simulink model "controllo_ss_PP_Luenberger"  (R2023b)
settings: Solver=VariableStepAuto  StartTime=0.0  StopTime=5  RelTol=1e-3
values from neighbouring files (symbols this model uses):
  A_ob = A - L_kf*C    [LQ_KF.m]    (also in LQ_KF_version1.m; LQ_KF_version2.m; LQ_Luenberger.m = A - L*C; LQ_prova.m)
  B_ob = [ B - L_kf*D, L_kf]    [LQ_KF.m]    (also in LQ_KF_version1.m; LQ_KF_version2.m; LQ_Luenberger.m = [ B - L*D, L]; LQ_prova.m)
  C_ob = eye(n)    [LQ_KF.m]    (also in LQ_KF_version1.m; LQ_KF_version2.m; LQ_Luenberger.m; LQ_prova.m)
  D_ob = zeros(n, m+p)    [LQ_KF.m]    (also in LQ_KF_version1.m; LQ_KF_version2.m; LQ_Luenberger.m; LQ_prova.m)
  Ken_eta = K(:, 4)    [LQ_KF.m]    (also in LQ_KF_version1.m; LQ_KF_version2.m = Ken(:, n+1:end); LQ_Luenberger.m; LQ_prova.m = Ken(:, n+1:end))
  Ken_x = K(:, 1:3)    [LQ_KF.m]    (also in LQ_KF_version1.m; LQ_KF_version2.m = Ken(:, 1:n); LQ_Luenberger.m; LQ_prova.m = Ken(:, 1:n))
undefined symbols (not defined in the file or in its folder): A, B, C, D, x1_eq0, x2_eq0
libraries: SignalEditorBlockLib x1
settings Model: Creator=Pronto all'uso  LastModifiedBy=lollo

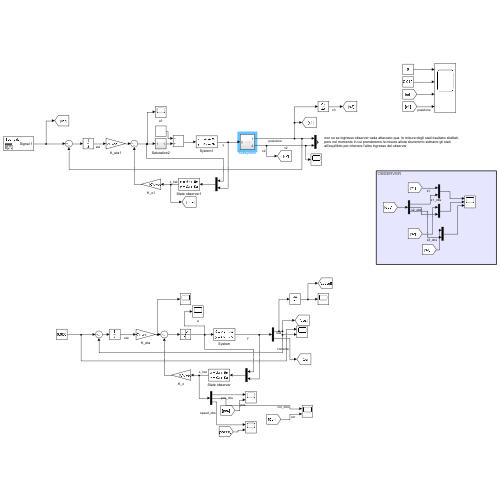
[thumbnail: Simulink's stored preview of the top-level diagram]
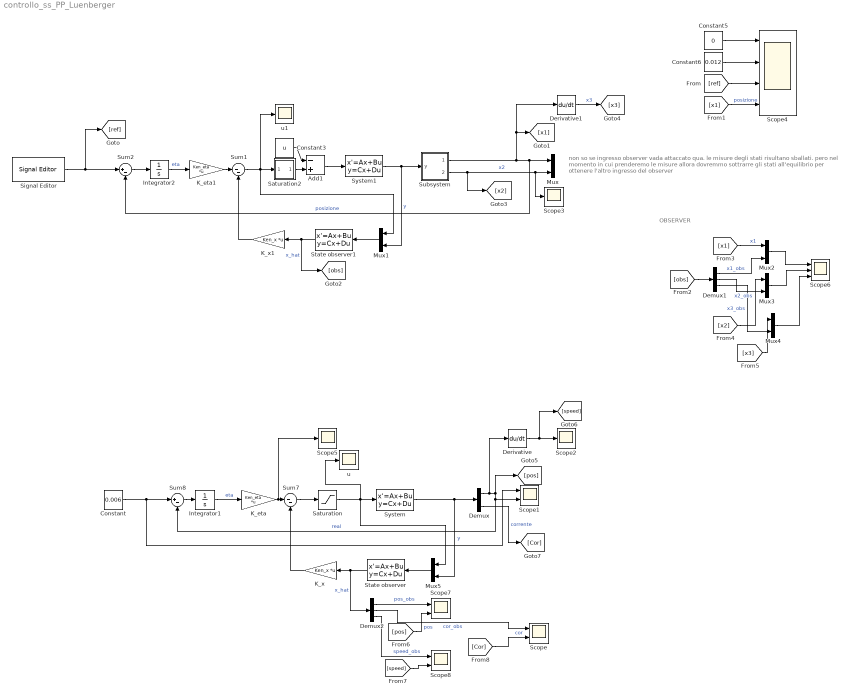
== system controllo_ss_PP_Luenberger ==
  note: OBSERVER
  note: non so se ingresso observer vada attaccato qua. le misure degli stati risultano sballati. pero nel momento in cui prenderemo le misure allora dovremmo sottrarre gli stati all'equilibrio per ottenere l'altro ingresso del observer
  Add1 : Sum  Inputs=-+
  Constant : Constant  Value=0.006
  Constant3 : Constant  Value=u
  Constant5 : Constant  Value=0
  Constant6 : Constant  Value=0.012
  Demux : Demux  Outputs=2
  Demux1 : Demux  Outputs=3
  Demux2 : Demux  Outputs=3
  Derivative : Derivative
  Derivative1 : Derivative
  Integrator1 : Integrator
  Integrator2 : Integrator
  K_eta : Gain  Gain=Ken_eta  Multiplication=Matrix(K*u) (u vector)
  K_eta1 : Gain  Gain=Ken_eta  Multiplication=Matrix(K*u) (u vector)
  K_x : Gain  Gain=Ken_x  Multiplication=Matrix(K*u) (u vector)
  K_x1 : Gain  Gain=Ken_x  Multiplication=Matrix(K*u) (u vector)
  Mux{,1..5} (6 alike) : Mux  Inputs=2
  Saturation : Saturate  UpperLimit=23  LowerLimit=-23
  Saturation2 : Subsystem
  Scope{,1,7..8} (4 alike) : Scope  NumInputPorts=2
  Scope2 : Scope
  Scope3 : Scope
  Scope4 : Scope  NumInputPorts=4
  Scope5 : Scope
  Scope6 : Scope  NumInputPorts=3
  Signal Editor : SignalEditorBlockLib/Signal Editor  FileName=input_signal.mat  ActiveScenario=Scenario  ActiveSignal=Signal 1  IsBus=off  OutputBusObjectStr=Bus: BusObject  SampleTime=0  Interpolate=off  ZeroCross=off  OutputAfterFinalValue=Setting to zero  Unit=inherit  PreserveSignalName=on  ApplySigPropsToAllScenarios=on  ApplySigPropsToAllSignals=off
  State observer : StateSpace  A=A_ob  B=B_ob  C=C_ob  D=D_ob  InitialCondition=[0.002;0;0]  ParameterTunability=Unconstrained
  State observer1 : StateSpace  A=A_ob  B=B_ob  C=C_ob  D=D_ob  InitialCondition=[0.002;0;0]  ParameterTunability=Unconstrained
  Subsystem : Subsystem
  Sum1 : Sum  Inputs=|--
  Sum2 : Sum  Inputs=|+-
  Sum7 : Sum  Inputs=|--
  Sum8 : Sum  Inputs=|+-
  System : StateSpace  A=A  B=B  C=C  D=D  InitialCondition=[0; 0;0]  ParameterTunability=Unconstrained
  System1 : StateSpace  A=A  B=B  C=C  D=D  InitialCondition=[0; 0;0]  ParameterTunability=Unconstrained
  u : Scope
  u1 : Scope
  wires:
  Integrator1/1 -> K_eta/1  "eta"
  K_x/1 -> Sum7/2
  Sum8/1 -> Integrator1/1
  K_eta/1 -> Scope5/1, Sum7/1
  System/1 -> Demux/1, Mux5/2  "y"
  State observer/1 -> Demux2/1, K_x/1  "x_hat"
  Mux5/1 -> State observer/1
  Demux/1 -> Derivative/1, [pos], Scope1/2, Sum8/2  "real"
  Demux/2 -> [Cor]  "corrente"
  Constant/1 -> Scope1/1, Sum8/1
  Sum7/1 -> Saturation/1
  Saturation/1 -> Mux5/1, u/1, System/1
  Derivative/1 -> [speed], Scope2/1
  State observer1/1 -> [obs], K_x1/1  "x_hat"
  Sum2/1 -> Integrator2/1
  Integrator2/1 -> K_eta1/1  "eta"
  Sum1/1 -> u1/1, Saturation2/1(In1), Mux1/1
  K_eta1/1 -> Sum1/1
  K_x1/1 -> Sum1/2
  Signal Editor/1 -> [ref], Sum2/1
  Mux1/1 -> State observer1/1
  [ref] -> Scope4/3
  Add1/1 -> System1/1
  Constant3/1 -> Add1/1
  Constant5/1 -> Scope4/1
  Constant6/1 -> Scope4/2
  Saturation2/1(Out1) -> Add1/2
  Subsystem/2(Out2) -> [x2], Mux/2, Scope3/1  "x2"
  Subsystem/1(Out1) -> [x1], Derivative1/1, Mux/1, Sum2/2  "posizione"
  System1/1 -> Mux1/2, Subsystem/1(y)  "y"
  [x1] -> Scope4/4  "posizione"
  [obs] -> Demux1/1
  [x1] -> Mux2/1  "x1"
  Demux1/1 -> Mux2/2  "x1_obs"
  Demux1/2 -> Mux3/2  "x2_obs"
  [x2] -> Mux3/1
  Mux3/1 -> Scope6/2
  Mux2/1 -> Scope6/1
  Demux1/3 -> Mux4/2  "x3_obs"
  Derivative1/1 -> [x3]  "x3"
  [x3] -> Mux4/1
  Mux4/1 -> Scope6/3
  Demux2/1 -> Scope7/1  "pos_obs"
  [pos] -> Scope7/2  "pos"
  Demux2/3 -> Scope8/1  "speed_obs"
  [speed] -> Scope8/2
  Demux2/2 -> Scope/1  "cor_obs"
  [Cor] -> Scope/2  "cor"

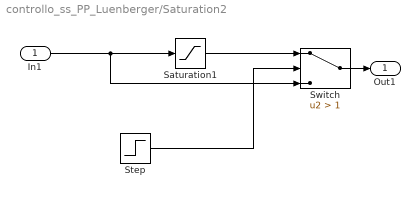
== system controllo_ss_PP_Luenberger/Saturation2 ==
  In1 : Inport
  Saturation1 : Saturate  UpperLimit=23  LowerLimit=-23
  Step : Step  SampleTime=0
  Switch : Switch  Criteria=u2 > Threshold  Threshold=1  SaturateOnIntegerOverflow=off  InputSameDT=off
  Out1 : Outport
  wires:
  Saturation1/1 -> Switch/1
  In1/1 -> Switch/3, Saturation1/1
  Switch/1 -> Out1/1
  Step/1 -> Switch/2

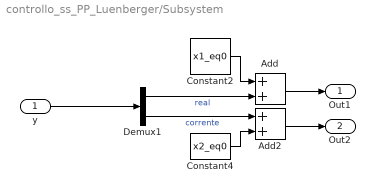
== system controllo_ss_PP_Luenberger/Subsystem ==
  y : Inport
  Add : Sum
  Add2 : Sum
  Constant2 : Constant  Value=x1_eq0
  Constant4 : Constant  Value=x2_eq0
  Demux1 : Demux  Outputs=2
  Out1 : Outport
  Out2 : Outport  Port=2
  wires:
  Add/1 -> Out1/1
  Constant4/1 -> Add2/2
  Constant2/1 -> Add/1
  Demux1/1 -> Add/2  "real"
  Add2/1 -> Out2/1
  Demux1/2 -> Add2/1  "corrente"
  y/1 -> Demux1/1
